simulink model "orbitEOM_o_e_graph"  (R2022b)
settings: Solver=FixedStepAuto  StartTime=0.0  StopTime=tstop  FixedStep=maxstep  MaxStep=maxstep  RelTol=1e-3  EnableMultiTasking=on
values from neighbouring files (symbols this model uses):
  a_set = opt_cooef(2:end)    [evaluate_cost_orb_elem.m]    (also in multi_plot.m = opt_cooef_3(2:end))
  m_dot = 0.04    [mars_optimized.m]    (also in mars_set_up.m; multi_plot.m = m_dot_3)
  mass_init = 250000    [mars_optimized.m]    (also in mars_set_up.m)
  MuS = 1.32747e20    (= 1.32747e+20)    [cost_function_orb_elem.m]    (also in mars_optimized.m; mars_set_up.m)
  r0 = (rs)*[1 0 0].'    [mars_optimized.m]    (also in mars_set_up.m)
  t_flip = opt_cooef(1)    [evaluate_cost_orb_elem.m]    (also in multi_plot.m = opt_cooef_3(1))
  thrust = 0.019*mass_init*9.81    (= 46597.5)    [mars_optimized.m]    (also in mars_set_up.m; multi_plot.m = thrust_3)
  v0 = sqrt(MuS/norm(r0))*[0 1 0].'    [mars_optimized.m]    (also in mars_set_up.m)
settings Model: Creator=Mason  LastModifiedBy=erikpayton
settings SolverCC: AlgebraicLoopSolver=TrustRegion
settings DataIOCC: LimitDataPoints=on  SaveFormat=Array  SignalLoggingSaveFormat=ModelDataLogs  ReturnWorkspaceOutputs=off  SignalLoggingName=sigsOut
settings OptimizationCC: ExpressionDepthLimit=2147483647  InitFltsAndDblsToZero=on  LifeSpan=inf
settings DebuggingCC: SaveWithParameterizedLinksMsg=none  UnderspecifiedInitializationDetection=Classic  MergeDetectMultiDrivingBlocksExec=none  SignalResolutionControl=TryResolveAllWithWarning  MultiTaskDSMMsg=warning  MultiTaskCondExecSysMsg=none  FcnCallInpInsideContextMsg=warning  UnconnectedInputMsg=warning  UnconnectedOutputMsg=warning  UnconnectedLineMsg=warning  StateNameClashWarn=warning  SFUnexpectedBacktrackingDiag=warning  SFNoUnconditionalDefaultTransitionDiag=warning  SFExecutionAtInitializationDiag=none  SFMachineParentedDataDiag=warning  ArithmeticOperatorsInVariantConditions=warning
settings HardwareCC: ProdBitPerPointer=32  ProdBitPerSizeT=32  ProdBitPerPtrDiffT=32  ProdLargestAtomicFloat=None  ProdIntDivRoundTo=Undefined  ProdEndianess=Unspecified  ProdWordSize=32  ProdHWDeviceType=32-bit Generic  TargetUnknown=on
settings ModelReferenceCC: EnableRefExpFcnMdlSchedulingChecks=on  PropagateSignalLabelsOutOfModel=off
settings SFSimCC: SimUseLocalCustomCode=off  CustomCodeUndefinedFunction=UseInterfaceOnly
settings RTWCC: RTWUseLocalCustomCode=off  DLArmComputeVersion=19.05
settings CodeAppCC: StateflowObjectComments=on
settings GRTTargetCC: TargetFcnLib=ansi_tfl_tmw.mat  TargetLangStandard=C89/C90 (ANSI)  CombineOutputUpdateFcns=off  GRTInterface=on
settings ConfigComp: CovMetricSettings=dw  CovSaveCumulativeToWorkspaceVar=on  CovSaveSingleToWorkspaceVar=on  CovExternalEMLEnable=off
settings SimscapeCC: SimscapeNormalizeSystem=off

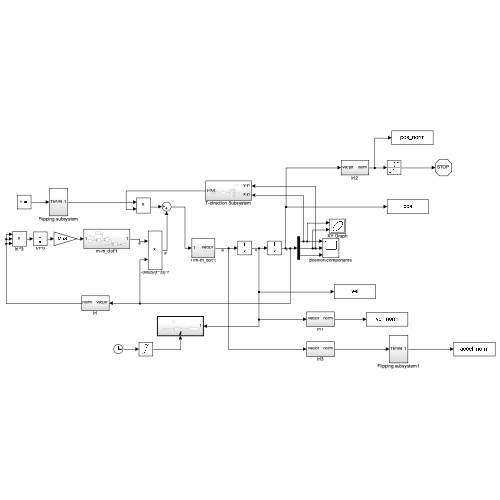
[thumbnail: Simulink's stored preview of the top-level diagram]
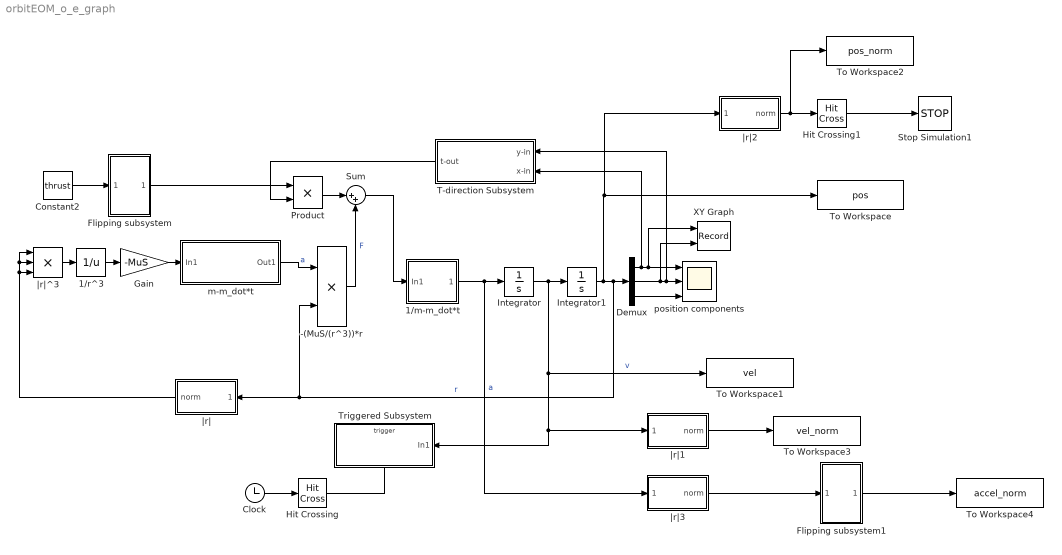
== system orbitEOM_o_e_graph ==
  -(MuS/(r^3))*r : Product
  1/m-m_dot*t : Subsystem
  1/r^3 : Math  Operator=reciprocal
  Clock : Clock
  Constant2 : Constant  Value=thrust
  Demux : Demux  Outputs=3
      settings: DisplayOption=none
  Flipping subsystem : Subsystem
  Flipping subsystem1 : Subsystem
  Gain : Gain  Gain=-MuS  SaturateOnIntegerOverflow=on  OutDataTypeStr=Inherit: Same as input  ParamDataTypeStr=Inherit: Same as input
  Hit Crossing : HitCross  HitCrossingOffset=t_flip  HitCrossingDirection=rising
  Hit Crossing1 : HitCross  HitCrossingOffset=d_o  HitCrossingDirection=rising
  Integrator : Integrator  InitialCondition=v0
  Integrator1 : Integrator  InitialCondition=r0
  Product : Product
  Stop Simulation1 : Stop
  Sum : Sum  Inputs=|++
  T-direction Subsystem : Subsystem
  To Workspace : ToWorkspace  VariableName=pos  SaveFormat=Timeseries  SampleTime=-1
  To Workspace1 : ToWorkspace  VariableName=vel  SampleTime=-1
  To Workspace2 : ToWorkspace  VariableName=pos_norm  SaveFormat=Timeseries  SampleTime=-1
  To Workspace3 : ToWorkspace  VariableName=vel_norm  SaveFormat=Timeseries  SampleTime=-1
  To Workspace4 : ToWorkspace  VariableName=accel_norm  SaveFormat=Timeseries  SampleTime=-1
  Triggered Subsystem : Subsystem  TreatAsAtomicUnit=on
  XY Graph : Record  FileSettingsInternal="{\"entries\":[{\"content\":{\"excelSettings\":{\"content\":{},\"type\":\"Streamout.ExcelSettings\"}},\"type\":\"Streamout.FileSettingStorage\",\"uuid\":\"ff7e06af-6e21-4bd0-9966-7a4d89266818\"}],\"packageUris\":[\"http://schema.mathworks.com/mf0/streamout_blocks/R2020a\"],\"version\":\"1.0\"}"  Layout=[1 1]  SignalsInternal="{\"entries\":[{\"content\":{\"signals\":[{\"content\":{\"blockPath\":[\"orbitEOM_o_e_graph/XY Graph\"],\"channel\":[],\"dimensions\":[1],\"domain\":\"orbitEOM_o_e_graph/XY Graph\",\"lineColor\":\"#a2142f\",\"plots\":[1],\"port\":1,\"sid\":[\"\"],\"signalID\":75897,\"signalName\":\"Demux:1\"},\"type\":\"RecordBlkView.Signal\",\"uuid\":\"e02dfef0-b3ca-4bda-9eec-72397f5a5bda\"},{\"content\":{\"blockPath\":[\"orbitEOM_o_e_graph/XY Graph\"],\"channel\":[],\"dimensions\":[1],\"domain\":\"orbitEOM_o_e_graph/XY Graph\",\"lineColor\":\"#139fff\",\"plots\":[1],\"port\":2,\"sid\":[\"\"],\"signalID\":75901,\"signalName\":\"Demux:2\"},\"type\":\"RecordBlkView.Signal\",\"uuid\":\"b7d16e6c-c502-4a38-9da5-6f9615b79b83\"}]},\"type\":\"RecordBlkView.InputSignals\",\"uuid\":\"c905ae1e-553d-40d9-8e89-6a9bf88f0ab8\"}],\"packageUris\":[\"http://schema.mathworks.com/mf0/streamout_blocks/R2020a\"],\"version\":\"1.0\"}"  VisualizationBindings="{\"xyplotplugin\":{\"info\":[{\"series\":[{\"bindingParametersList\":[{\"parameter\":\"X-Axis\",\"signalID\":75897,\"signalName\":\"Demux:1\"},{\"parameter\":\"Y-Axis\",\"signalID\":75901,\"signalName\":\"Demux:2\"}],\"seriesID\":42219}],\"subplotID\":1}]}}"  CompatibilityTag=XY
  m-m_dot*t : Subsystem
  position components : Scope  NumInputPorts=3
  |r| : Subsystem
  |r|1 : Subsystem
  |r|2 : Subsystem
  |r|3 : Subsystem
  |r|^3 : Product  Inputs=3
  wires:
  Integrator1/1 -> |r|2/1(vector), To Workspace/1, -(MuS/(r^3))*r/2, |r|/1(vector), Demux/1  "r"
  Integrator/1 -> |r|1/1(vector), Triggered Subsystem/1(In1), To Workspace1/1, Integrator1/1  "v"
  Demux/3 -> position components/3
  Demux/1 -> T-direction Subsystem/2(x-in), XY Graph/1, position components/1
  Demux/2 -> T-direction Subsystem/1(y-in), position components/2, XY Graph/2
  1/m-m_dot*t/1(vector) -> |r|3/1(vector), Integrator/1  "a"
  1/r^3/1 -> Gain/1
  -(MuS/(r^3))*r/1 -> Sum/2  "F"
  |r|^3/1 -> 1/r^3/1
  |r|/1(norm) -> |r|^3/2, |r|^3/1, |r|^3/3
  Gain/1 -> m-m_dot*t/1(In1)
  m-m_dot*t/1(Out1) -> -(MuS/(r^3))*r/1  "a"
  Sum/1 -> 1/m-m_dot*t/1(In1)
  Product/1 -> Sum/1
  T-direction Subsystem/1(t-out) -> Product/2
  |r|2/1(norm) -> To Workspace2/1, Hit Crossing1/1
  Hit Crossing1/1 -> Stop Simulation1/1
  Flipping subsystem/1(Out1) -> Product/1
  Constant2/1 -> Flipping subsystem/1(Thrust)
  Clock/1 -> Hit Crossing/1
  Hit Crossing/1 -> Triggered Subsystem/Trigger
  |r|3/1(norm) -> Flipping subsystem1/1(Thrust)
  |r|1/1(norm) -> To Workspace3/1
  Flipping subsystem1/1(Out1) -> To Workspace4/1

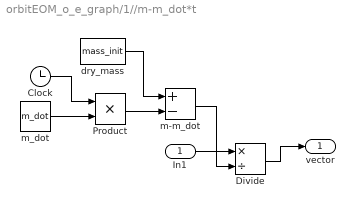
== system orbitEOM_o_e_graph/1//m-m_dot*t ==
  In1 : Inport
  Clock : Clock
  Divide : Product  Inputs=*/
  Product : Product
  dry_mass : Constant  Value=mass_init
  m-m_dot : Sum  Inputs=+-
  m_dot : Constant  Value=m_dot
  vector : Outport
  wires:
  Divide/1 -> vector/1
  In1/1 -> Divide/1
  Product/1 -> m-m_dot/2
  dry_mass/1 -> m-m_dot/1
  m-m_dot/1 -> Divide/2
  m_dot/1 -> Product/2
  Clock/1 -> Product/1

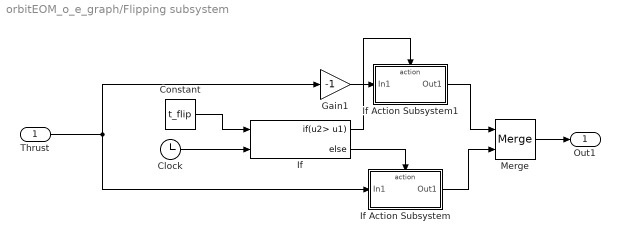
== system orbitEOM_o_e_graph/Flipping subsystem ==
  Thrust : Inport
  Clock : Clock
  Constant : Constant  Value=t_flip
  Gain1 : Gain  Gain=-1
  If : If  NumInputs=2  IfExpression=u2> u1
  If Action Subsystem : Subsystem  TreatAsAtomicUnit=on
  If Action Subsystem1 : Subsystem  TreatAsAtomicUnit=on
  Merge : Merge
  Out1 : Outport
  wires:
  If/2 -> If Action Subsystem/Action
  Thrust/1 -> If Action Subsystem/1(In1), Gain1/1
  Merge/1 -> Out1/1
  If Action Subsystem1/1(Out1) -> Merge/1
  Constant/1 -> If/1
  If Action Subsystem/1(Out1) -> Merge/2
  Gain1/1 -> If Action Subsystem1/1(In1)
  If/1 -> If Action Subsystem1/Action
  Clock/1 -> If/2

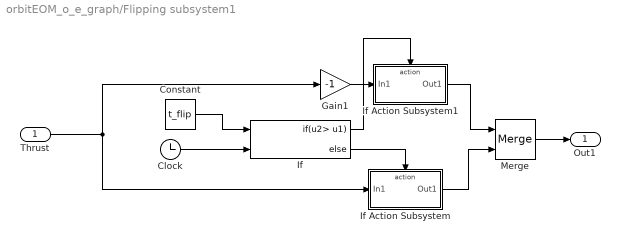
== system orbitEOM_o_e_graph/Flipping subsystem1 ==
  Thrust : Inport
  Clock : Clock
  Constant : Constant  Value=t_flip
  Gain1 : Gain  Gain=-1
  If : If  NumInputs=2  IfExpression=u2> u1
  If Action Subsystem : Subsystem  TreatAsAtomicUnit=on
  If Action Subsystem1 : Subsystem  TreatAsAtomicUnit=on
  Merge : Merge
  Out1 : Outport
  wires:
  If/2 -> If Action Subsystem/Action
  Thrust/1 -> If Action Subsystem/1(In1), Gain1/1
  Merge/1 -> Out1/1
  If Action Subsystem1/1(Out1) -> Merge/1
  Constant/1 -> If/1
  If Action Subsystem/1(Out1) -> Merge/2
  Gain1/1 -> If Action Subsystem1/1(In1)
  If/1 -> If Action Subsystem1/Action
  Clock/1 -> If/2

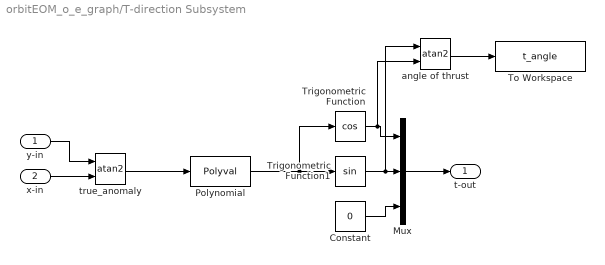
== system orbitEOM_o_e_graph/T-direction Subsystem ==
  y-in : Inport
  x-in : Inport  Port=2
  Constant : Constant  Value=0
  Mux : Mux  Inputs=3
  Polynomial : Polyval  Coefs=a_set
  To Workspace : ToWorkspace  VariableName=t_angle  SampleTime=-1
      settings: Save2DSignal=2-D array (concatenate along first dimension)
  Trigonometric Function : Trigonometry  Operator=cos
  Trigonometric Function1 : Trigonometry
  angle of thrust : Trigonometry  Operator=atan2
  true_anomaly : Trigonometry  Operator=atan2
  t-out : Outport
  wires:
  Trigonometric Function1/1 -> angle of thrust/1, Mux/2
  Constant/1 -> Mux/3
  Trigonometric Function/1 -> angle of thrust/2, Mux/1
  Mux/1 -> t-out/1
  Polynomial/1 -> Trigonometric Function1/1, Trigonometric Function/1
  true_anomaly/1 -> Polynomial/1
  x-in/1 -> true_anomaly/2
  y-in/1 -> true_anomaly/1
  angle of thrust/1 -> To Workspace/1

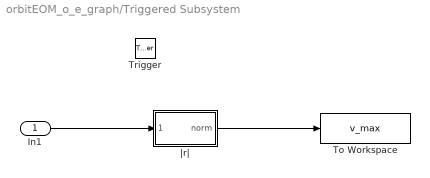
== system orbitEOM_o_e_graph/Triggered Subsystem ==
  In1 : Inport
  Trigger : TriggerPort  VariantControl=(inherit)
  To Workspace : ToWorkspace  VariableName=v_max  SampleTime=-1
  |r| : Subsystem
  wires:
  In1/1 -> |r|/1(vector)
  |r|/1(norm) -> To Workspace/1

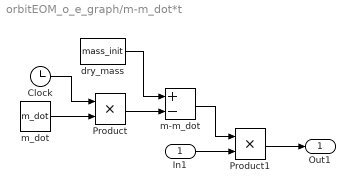
== system orbitEOM_o_e_graph/m-m_dot*t ==
  In1 : Inport
  Clock : Clock
  Product : Product
  Product1 : Product
  dry_mass : Constant  Value=mass_init
  m-m_dot : Sum  Inputs=+-
  m_dot : Constant  Value=m_dot
  Out1 : Outport
  wires:
  Product1/1 -> Out1/1
  In1/1 -> Product1/2
  Product/1 -> m-m_dot/2
  dry_mass/1 -> m-m_dot/1
  m-m_dot/1 -> Product1/1
  m_dot/1 -> Product/2
  Clock/1 -> Product/1

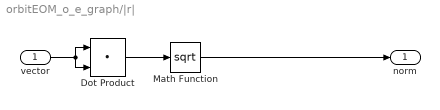
== system orbitEOM_o_e_graph/|r| ==
  vector : Inport
  Dot Product : DotProduct  OutDataTypeStr=Inherit: Inherit via internal rule
  Math Function : Math  Operator=sqrt  SignedPower=on
  norm : Outport  VectorParamsAs1DForOutWhenUnconnected=off
  wires:
  vector/1 -> Dot Product/1, Dot Product/2
  Dot Product/1 -> Math Function/1
  Math Function/1 -> norm/1

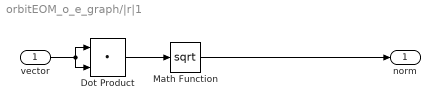
== system orbitEOM_o_e_graph/|r|1 ==
  vector : Inport
  Dot Product : DotProduct  OutDataTypeStr=Inherit: Inherit via internal rule
  Math Function : Math  Operator=sqrt  SignedPower=on
  norm : Outport  VectorParamsAs1DForOutWhenUnconnected=off
  wires:
  vector/1 -> Dot Product/1, Dot Product/2
  Dot Product/1 -> Math Function/1
  Math Function/1 -> norm/1

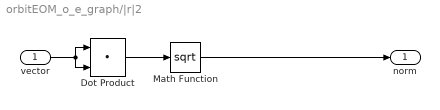
== system orbitEOM_o_e_graph/|r|2 ==
  vector : Inport
  Dot Product : DotProduct  OutDataTypeStr=Inherit: Inherit via internal rule
  Math Function : Math  Operator=sqrt  SignedPower=on
  norm : Outport  VectorParamsAs1DForOutWhenUnconnected=off
  wires:
  vector/1 -> Dot Product/1, Dot Product/2
  Dot Product/1 -> Math Function/1
  Math Function/1 -> norm/1

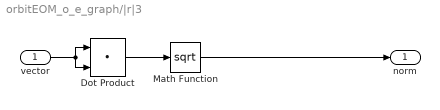
== system orbitEOM_o_e_graph/|r|3 ==
  vector : Inport
  Dot Product : DotProduct  OutDataTypeStr=Inherit: Inherit via internal rule
  Math Function : Math  Operator=sqrt  SignedPower=on
  norm : Outport  VectorParamsAs1DForOutWhenUnconnected=off
  wires:
  vector/1 -> Dot Product/1, Dot Product/2
  Dot Product/1 -> Math Function/1
  Math Function/1 -> norm/1

== system orbitEOM_o_e_graph/Flipping subsystem/If Action Subsystem ==
  In1 : Inport
  Action Port : ActionPort  ActionPortLabel=else
  Out1 : Outport
  wires:
  In1/1 -> Out1/1

== system orbitEOM_o_e_graph/Flipping subsystem/If Action Subsystem1 ==
  In1 : Inport
  Action Port : ActionPort  ActionPortLabel=if(u2> u1)
  Out1 : Outport
  wires:
  In1/1 -> Out1/1

== system orbitEOM_o_e_graph/Flipping subsystem1/If Action Subsystem ==
  In1 : Inport
  Action Port : ActionPort  ActionPortLabel=else
  Out1 : Outport
  wires:
  In1/1 -> Out1/1

== system orbitEOM_o_e_graph/Flipping subsystem1/If Action Subsystem1 ==
  In1 : Inport
  Action Port : ActionPort  ActionPortLabel=if(u2> u1)
  Out1 : Outport
  wires:
  In1/1 -> Out1/1

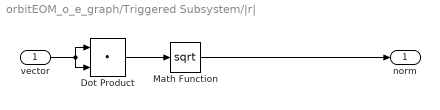
== system orbitEOM_o_e_graph/Triggered Subsystem/|r| ==
  vector : Inport
  Dot Product : DotProduct  OutDataTypeStr=Inherit: Inherit via internal rule
  Math Function : Math  Operator=sqrt  SignedPower=on
  norm : Outport  VectorParamsAs1DForOutWhenUnconnected=off
  wires:
  vector/1 -> Dot Product/1, Dot Product/2
  Dot Product/1 -> Math Function/1
  Math Function/1 -> norm/1
